simulink model "TCLab_model"  (R2022b)
settings: Solver=VariableStepAuto  StartTime=0.0  StopTime=10.0  RelTol=1e-3
values from neighbouring files (symbols this model uses):
  A = 0.001    [Variaveis.mat]    (also in lab1_2.m = 8; lab1_3.m = 8; tclabsim.m)
  alfa = 0.0131    [Variaveis.mat]    (also in tclabsim.m = p(2))
  Boltzman = 5.67e-08    [Variaveis.mat]    (also in tclabsim.m)
  Cp = 500    [Variaveis.mat]    (also in tclabsim.m)
  epsilon = 0.9    [Variaveis.mat]    (also in tclabsim.m)
  m = 0.004    [Variaveis.mat]    (also in tclabsim.m)
  Ta = 296.15    [Variaveis.mat]    (also in tclabsim.m = x0 + 272.15)
  tao = 21.1    [Variaveis.mat]    (also in tclabsim.m = p(3))
  U = 4.4    [Variaveis.mat]    (also in tclabsim.m = p(1); untitled.m = linspace(4.38381, 8.70219, MAX))
settings Model: Creator=wonebone  LastModifiedBy=wonebone

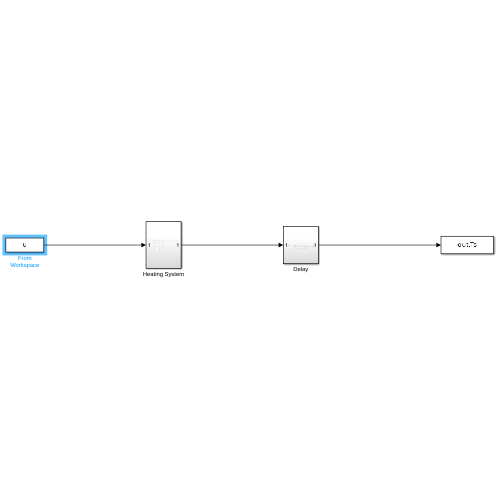
[thumbnail: Simulink's stored preview of the top-level diagram]
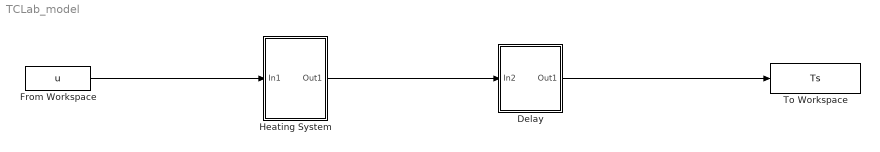
== system TCLab_model ==
  Delay : Subsystem
  From Workspace : FromWorkspace  VariableName=u
  Heating System : Subsystem
  To Workspace : ToWorkspace  VariableName=Ts  SaveFormat=Timeseries  SampleTime=-1
  wires:
  From Workspace/1 -> Heating System/1(In1)
  Heating System/1(Out1) -> Delay/1(In2)
  Delay/1(Out1) -> To Workspace/1

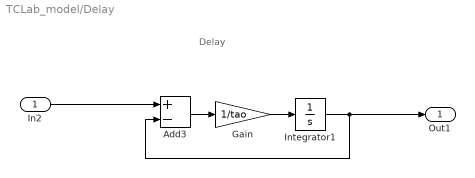
== system TCLab_model/Delay ==
  note: Delay
  In2 : Inport
  Add3 : Sum  Inputs=+-
  Gain : Gain  Gain=1/tao
  Integrator1 : Integrator  InitialCondition=Ta
  Out1 : Outport
  wires:
  Integrator1/1 -> Add3/2, Out1/1
  In2/1 -> Add3/1
  Add3/1 -> Gain/1
  Gain/1 -> Integrator1/1

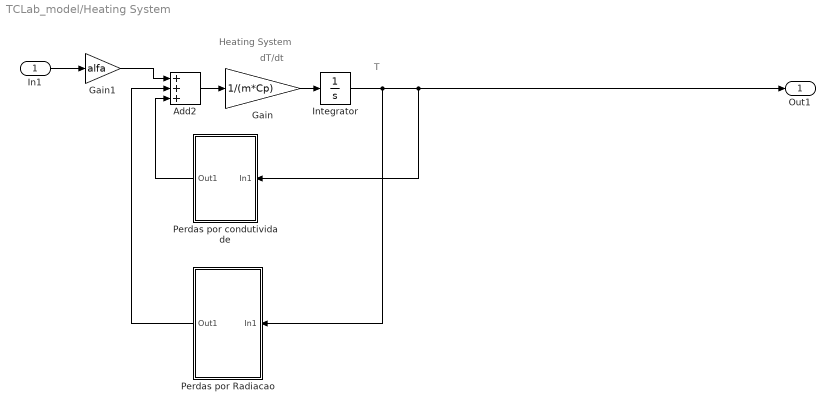
== system TCLab_model/Heating System ==
  note: Heating System
  note: T
  note: dT/dt
  In1 : Inport
  Add2 : Sum  Inputs=+++
  Gain : Gain  Gain=1/(m*Cp)
  Gain1 : Gain  Gain=alfa
  Integrator : Integrator  InitialCondition=Ta
  Perdas por Radiacao : Subsystem
  Perdas por condutividade : Subsystem
  Out1 : Outport
  wires:
  Gain/1 -> Integrator/1
  Integrator/1 -> Perdas por Radiacao/1(In1), Perdas por condutividade/1(In1), Out1/1
  Add2/1 -> Gain/1
  Gain1/1 -> Add2/1
  In1/1 -> Gain1/1
  Perdas por condutividade/1(Out1) -> Add2/3
  Perdas por Radiacao/1(Out1) -> Add2/2

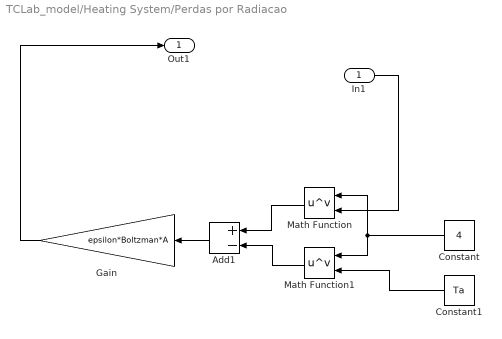
== system TCLab_model/Heating System/Perdas por Radiacao ==
  In1 : Inport
  Add1 : Sum  Inputs=+-
  Constant : Constant  Value=4
  Constant1 : Constant  Value=Ta
  Gain : Gain  Gain=epsilon*Boltzman*A
  Math Function : Math  Operator=pow
  Math Function1 : Math  Operator=pow
  Out1 : Outport
  wires:
  Add1/1 -> Gain/1
  Gain/1 -> Out1/1
  In1/1 -> Math Function/2
  Constant/1 -> Math Function1/1, Math Function/1
  Math Function/1 -> Add1/1
  Math Function1/1 -> Add1/2
  Constant1/1 -> Math Function1/2

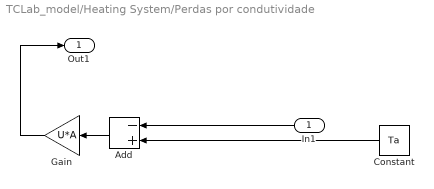
== system TCLab_model/Heating System/Perdas por condutividade ==
  In1 : Inport
  Add : Sum  Inputs=-+
  Constant : Constant  Value=Ta
  Gain : Gain  Gain=U*A
  Out1 : Outport
  wires:
  Add/1 -> Gain/1
  In1/1 -> Add/1
  Gain/1 -> Out1/1
  Constant/1 -> Add/2
